simulink model "DischargeC21"  (R2020a)
settings: Solver=FixedStepAuto  StartTime=0.0  StopTime=10.0  FixedStep=1e-3  RelTol=1e-3  EnableMultiTasking=on
undefined symbols (not defined in the file): D10, D4, D7, PTB23, PTC3, PTD0
libraries: frdmk64flib x3
settings Model: ExtModeTrigDuration=5  Creator=WinnieTrandinh  LastModifiedBy=WinnieTrandinh
settings OptimizationCC: EnhancedBackFolding=on  PassReuseOutputArgsAs=Individual arguments  ZeroExternalMemoryAtStartup=off  ZeroInternalMemoryAtStartup=off  MaxStackSize=64  OptimizeBlockOrder=speed  DifferentSizesBufferReuse=on  OptimizationCustomize=off  EfficientTunableParamExpr=on
settings DebuggingCC: ParameterTunabilityLossMsg=error
settings HardwareCC: ProdBitPerPointer=32  ProdBitPerSizeT=32  ProdBitPerPtrDiffT=32  ProdLargestAtomicInteger=Long  ProdLargestAtomicFloat=Double  ProdWordSize=32  ProdHWDeviceType=ARM Compatible->ARM Cortex
settings SFSimCC: MATLABDynamicMemAlloc=off
settings RTWCC: SystemTargetFile=ert.tlc  HardwareBoard=NXP FRDM-K64F  TemplateMakefile=ert_default_tmf  Toolchain=GNU Tools for ARM Embedded Processors
settings CodeAppCC: ForceParamTrailComments=on  IgnoreCustomStorageClasses=off  OperatorAnnotations=on  SimulinkDataObjDesc=on  SFDataObjDesc=on  InsertBlockDesc=on

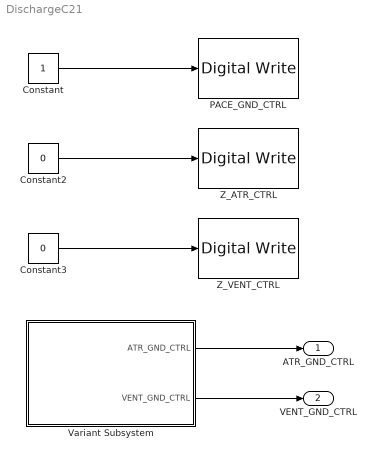
== system DischargeC21 ==
  Constant : Constant
  Constant2 : Constant  Value=0
  Constant3 : Constant  Value=0
  PACE_GND_CTRL : frdmk64flib/Digital Write  Whichpin=PTD0 (D10)
  Variant Subsystem : Subsystem  Variant=on
  Z_ATR_CTRL : frdmk64flib/Digital Write  Whichpin=PTB23 (D4)
  Z_VENT_CTRL : frdmk64flib/Digital Write  Whichpin=PTC3 (D7)
  ATR_GND_CTRL : Outport
  VENT_GND_CTRL : Outport  Port=2
  wires:
  Constant3/1 -> Z_VENT_CTRL/1
  Constant2/1 -> Z_ATR_CTRL/1
  Constant/1 -> PACE_GND_CTRL/1
  Variant Subsystem/1(ATR_GND_CTRL) -> ATR_GND_CTRL/1
  Variant Subsystem/2(VENT_GND_CTRL) -> VENT_GND_CTRL/1

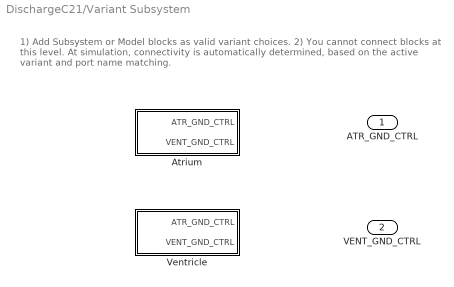
== system DischargeC21/Variant Subsystem ==
  note: 1) Add Subsystem or Model blocks as valid variant choices.
      | 2) You cannot connect blocks at this level. At simulation, connectivity is automatically
      | determined, based on the active variant and port name matching.
  Atrium : Subsystem  Priority=5  VariantControl=ATR_PACING
  Ventricle : Subsystem  Priority=5  VariantControl=VENT_PACING
  ATR_GND_CTRL : Outport
  VENT_GND_CTRL : Outport  Port=2

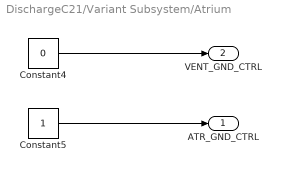
== system DischargeC21/Variant Subsystem/Atrium ==
  Constant4 : Constant  Value=0
  Constant5 : Constant
  ATR_GND_CTRL : Outport
  VENT_GND_CTRL : Outport  Port=2
  wires:
  Constant5/1 -> ATR_GND_CTRL/1
  Constant4/1 -> VENT_GND_CTRL/1

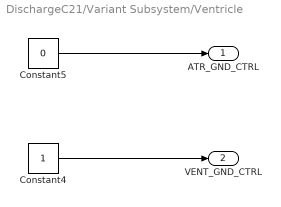
== system DischargeC21/Variant Subsystem/Ventricle ==
  Constant4 : Constant
  Constant5 : Constant  Value=0
  ATR_GND_CTRL : Outport
  VENT_GND_CTRL : Outport  Port=2
  wires:
  Constant4/1 -> VENT_GND_CTRL/1
  Constant5/1 -> ATR_GND_CTRL/1
